simulink model "Demo_EP_IdleRandMerg"  (R2014a)
settings: Solver=FixedStepDiscrete  SolverMode=SingleTasking  StartTime=0.0  StopTime=inf  FixedStep=0.01  RelTol=1e-3
PostLoadFcn:
  | h_RPStest = RPStest;
model workspace (MAT data in the model file):
  gtest = 0
undefined symbols (not defined in the file or in its folder): avert, avert_freq_factor, avert_gaze_dirs_chance, avert_gaze_duration_factor, avert_head_frequency_factor, avert_head_speed, BML, BML1, BML2, bmlsL, bmlsM, bodyBusyFlag, clock, emotion_amount_factor, faceBusyFlag, fileID, GAZE_WIN, gazing, mut_freq_factor, mutual_gaze_duration_factor, P, pose_cat_chance, pose_chanc_factor, pose_chance_factor, pose_change_flag, pose_frequency_factor, pose_lean, pose_lean_flag, pose_speed, pose_twitch, pr, serial, STATE_BEFORE, STATE_GO, STATE_OVER, STATE_READY, Stateflow
libraries: simulink x24, instrumentlib x6, lib_affectiveChar_behavior x3, realtime_pacer_lib x2, lib_affectiveChar_input x1
(part 4 of 7)

== system Demo_EP_IdleRandMerg/GazeFollowSubsystem/resetGazeTarget/createGazePawn/sendSBM ==
  In2 : Inport  OutDataTypeStr=double  PortDimensions=[1000 1]
  f : TriggerPort  TriggerType=function-call
      settings: CopyFcn=Stateflow.SLINSF.SimulinkMan.removeBlockPreDeleteFcn  PreDeleteFcn=Stateflow.SLINSF.SimulinkMan.unsafePredeleteFcn
  C++ S-Function2 : S-Function  FunctionName=yarpSendText_sfun  Parameters='/sim/out/smb8', '/SB/in/sbm'  EnableBusSupport=off
  wires:
  In2/1 -> C++ S-Function2/1

== system Demo_EP_IdleRandMerg/facialExpr/facialExprGen/emotionBMLsLoop ==
  Amounts : Inport
  AUs : Inport  Port=2
  i : Inport  Port=3  OutMin=1  OutDataTypeStr=double
  e : Inport  Port=4
  Delay : Delay  DelayLength=10  InitialCondition=10
  For Iterator : ForIterator  IterationSource=external
  bml1 : M-S-Function  FunctionName=yarpSendText2_sfun  Parameters='/sim/out/bml9', '/SB/in/bml'
  displayBMLs : MATLAB Function  TreatAsAtomicUnit=on
  loopInBmls : MATLAB Function  TreatAsAtomicUnit=on
  wires:
  AUs/1 -> loopInBmls/2(arrAU)
  Amounts/1 -> loopInBmls/3(eAmount)
  loopInBmls/1(arrBML) -> Delay/1, displayBMLs/3(bml)
  e/1 -> displayBMLs/1(e)
  Delay/1 -> bml1/1
  i/1 -> loopInBmls/1(i), displayBMLs/2(i)

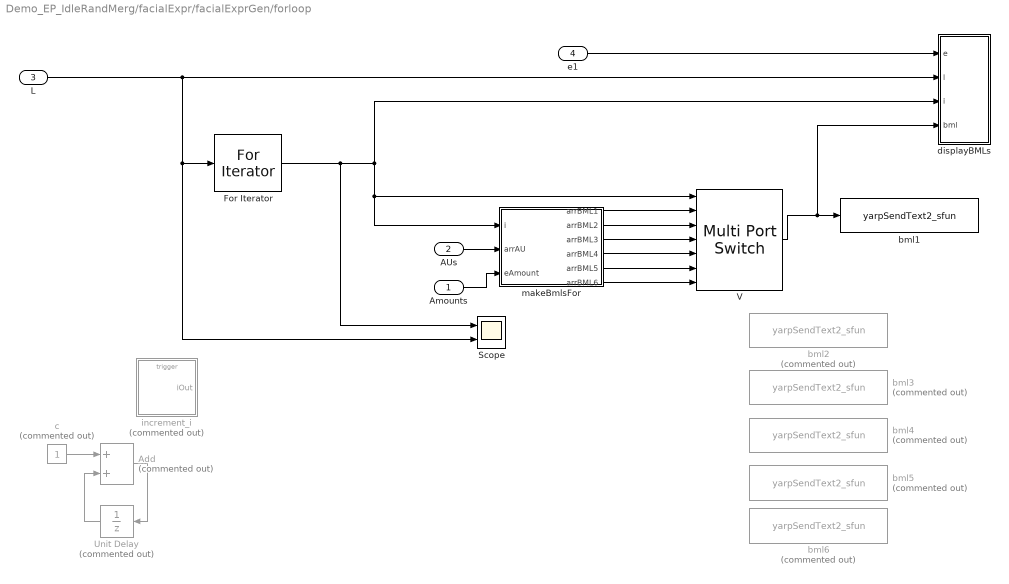
== system Demo_EP_IdleRandMerg/facialExpr/facialExprGen/forloop ==
  Amounts : Inport
  AUs : Inport  Port=2
  L : Inport  Port=3
  e1 : Inport  Port=4
  Add : Sum  Commented=on
  For Iterator : ForIterator  IterationSource=external  IterationVariableDataType=double
  Scope : Scope  NumInputPorts=2
      settings: YMin=3~3  YMax=3~3  SaveName=ScopeData7
  Unit Delay : UnitDelay  Commented=on  SampleTime=0.01
  V : MultiPortSwitch  Inputs=6
  bml1 : M-S-Function  FunctionName=yarpSendText2_sfun  Parameters='/sim/out/bml9', '/SB/in/bml'
  bml2 : M-S-Function  Commented=on  FunctionName=yarpSendText2_sfun  Parameters='/sim/out/bml10', '/SB/in/bml'
  bml3 : M-S-Function  Commented=on  FunctionName=yarpSendText2_sfun  Parameters='/sim/out/bml11', '/SB/in/bml'
  bml4 : M-S-Function  Commented=on  FunctionName=yarpSendText2_sfun  Parameters='/sim/out/bml12', '/SB/in/bml'
  bml5 : M-S-Function  Commented=on  FunctionName=yarpSendText2_sfun  Parameters='/sim/out/bml13', '/SB/in/bml'
  bml6 : M-S-Function  Commented=on  FunctionName=yarpSendText2_sfun  Parameters='/sim/out/bml14', '/SB/in/bml'
  c : Constant  Commented=on
  displayBMLs : MATLAB Function  TreatAsAtomicUnit=on
  increment_i : Subsystem  Commented=on
  makeBmlsFor : MATLAB Function  TreatAsAtomicUnit=on
  wires:
  L/1 -> Scope/2, For Iterator/1, displayBMLs/2(l)
  AUs/1 -> makeBmlsFor/2(arrAU)
  Amounts/1 -> makeBmlsFor/3(eAmount)
  e1/1 -> displayBMLs/1(e)
  Unit Delay/1 -> Add/2
  c/1 -> Add/1
  Add/1 -> Unit Delay/1
  For Iterator/1 -> Scope/1, V/1, makeBmlsFor/1(i), displayBMLs/3(i)
  V/1 -> displayBMLs/4(bml), bml1/1
  makeBmlsFor/1(arrBML1) -> V/2
  makeBmlsFor/2(arrBML2) -> V/3
  makeBmlsFor/3(arrBML3) -> V/4
  makeBmlsFor/4(arrBML4) -> V/5
  makeBmlsFor/5(arrBML5) -> V/6
  makeBmlsFor/6(arrBML6) -> V/7

== system Demo_EP_IdleRandMerg/facialExpr/facialExprGen/forloop1 ==
  Amounts : Inport
  AUs : Inport  Port=2
  L : Inport  Port=3
  e1 : Inport  Port=4
  Add : Sum  Commented=on
  Delay : Delay  DelayLength=50  InitialCondition=0
  For Iterator : ForIterator  IterationSource=external  IterationVariableDataType=double
  Scope : Scope  NumInputPorts=2
      settings: YMin=3~3  YMax=3~3  SaveName=ScopeData7
  Unit Delay : UnitDelay  Commented=on  SampleTime=0.01
  bml1 : M-S-Function  FunctionName=yarpSendText2_sfun  Parameters='/sim/out/bml9', '/SB/in/bml'
  c : Constant  Commented=on
  displayBMLs : MATLAB Function  TreatAsAtomicUnit=on
  increment_i : Subsystem  Commented=on
  makeBmls : MATLAB Function  TreatAsAtomicUnit=on
  wires:
  L/1 -> Scope/2, For Iterator/1, displayBMLs/2(l)
  AUs/1 -> makeBmls/2(arrAU)
  Amounts/1 -> makeBmls/3(eAmount)
  e1/1 -> displayBMLs/1(e)
  makeBmls/1(arrBML) -> Delay/1
  Unit Delay/1 -> Add/2
  c/1 -> Add/1
  Add/1 -> Unit Delay/1
  For Iterator/1 -> Scope/1, makeBmls/1(i), displayBMLs/3(i)
  Delay/1 -> displayBMLs/4(bml), bml1/1

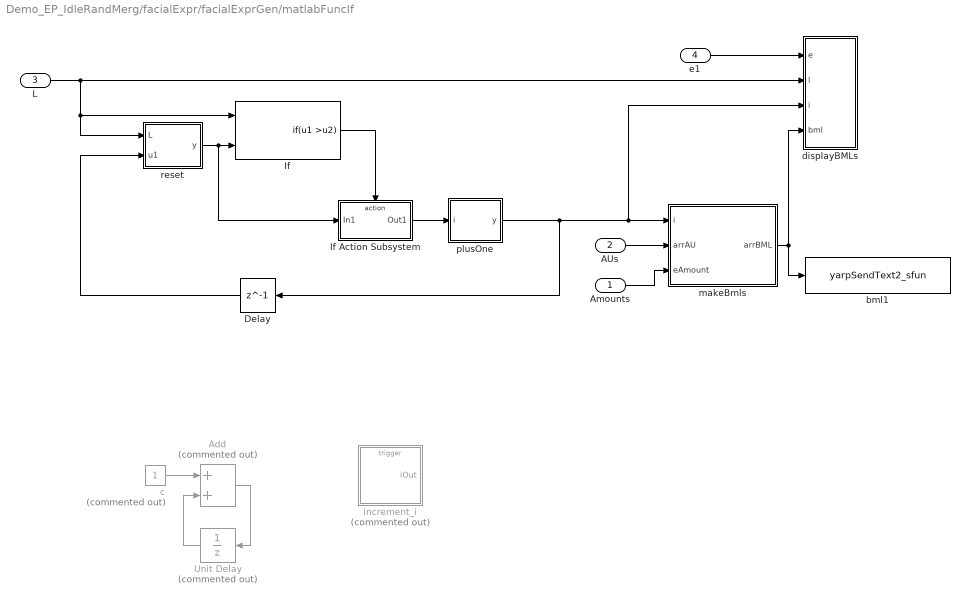
== system Demo_EP_IdleRandMerg/facialExpr/facialExprGen/matlabFuncIf ==
  Amounts : Inport
  AUs : Inport  Port=2
  L : Inport  Port=3
  e1 : Inport  Port=4
  Add : Sum  Commented=on
  Delay : Delay  DelayLength=1  InitialCondition=0
  If : If  NumInputs=2  IfExpression=u1 >u2  ShowElse=off
  If Action Subsystem : Subsystem  TreatAsAtomicUnit=on
  Unit Delay : UnitDelay  Commented=on  SampleTime=0.01
  bml1 : M-S-Function  FunctionName=yarpSendText2_sfun  Parameters='/sim/out/bml9', '/SB/in/bml'
  c : Constant  Commented=on
  displayBMLs : MATLAB Function  TreatAsAtomicUnit=on
  increment_i : Subsystem  Commented=on
  makeBmls : MATLAB Function  TreatAsAtomicUnit=on
  plusOne : MATLAB Function  TreatAsAtomicUnit=on
  reset : MATLAB Function  TreatAsAtomicUnit=on
  wires:
  L/1 -> reset/1(L), If/1, displayBMLs/2(l)
  AUs/1 -> makeBmls/2(arrAU)
  Amounts/1 -> makeBmls/3(eAmount)
  e1/1 -> displayBMLs/1(e)
  makeBmls/1(arrBML) -> displayBMLs/4(bml), bml1/1
  plusOne/1(y) -> Delay/1, displayBMLs/3(i), makeBmls/1(i)
  If/1 -> If Action Subsystem/Action
  Unit Delay/1 -> Add/2
  c/1 -> Add/1
  Add/1 -> Unit Delay/1
  If Action Subsystem/1(Out1) -> plusOne/1(i)
  Delay/1 -> reset/2(u1)
  reset/1(y) -> If Action Subsystem/1(In1), If/2

== system Demo_EP_IdleRandMerg/readGlove/normal glove/Normalize Index ==
  RawGlove : Inport
  Divide : Product  Inputs=*/  OutDataTypeStr=double  RndMeth=Nearest  InputSameDT=on
  Divide1 : Product  Inputs=**
  MinMax : Subsystem
  Range : Sum  Inputs=+-  OutDataTypeStr=double
  Ring1 : Constant  Value=100
  Subtract5 : Sum  Inputs=+-  OutDataTypeStr=double
  Norm100Out : Outport
  wires:
  MinMax/2(Max) -> Range/1
  Ring1/1 -> Divide1/2
  Subtract5/1 -> Divide/1
  MinMax/1(Min) -> Subtract5/2, Range/2
  RawGlove/1 -> Subtract5/1, MinMax/1(In1)
  Divide1/1 -> Norm100Out/1
  Divide/1 -> Divide1/1
  Range/1 -> Divide/2

== system Demo_EP_IdleRandMerg/readGlove/normal glove/Normalize Middle ==
  RawGlove : Inport
  Divide : Product  Inputs=*/  OutDataTypeStr=double  RndMeth=Nearest  InputSameDT=on
  Divide1 : Product  Inputs=**
  MinMax : Subsystem
  Range : Sum  Inputs=+-  OutDataTypeStr=double
  Ring1 : Constant  Value=100
  Subtract5 : Sum  Inputs=+-  OutDataTypeStr=double
  Norm100Out : Outport
  wires:
  MinMax/2(Max) -> Range/1
  Ring1/1 -> Divide1/2
  Subtract5/1 -> Divide/1
  MinMax/1(Min) -> Subtract5/2, Range/2
  RawGlove/1 -> Subtract5/1, MinMax/1(In1)
  Divide1/1 -> Norm100Out/1
  Divide/1 -> Divide1/1
  Range/1 -> Divide/2

== system Demo_EP_IdleRandMerg/readGlove/normal glove/Normalize Ring ==
  RawGlove : Inport
  Divide : Product  Inputs=*/  OutDataTypeStr=double  RndMeth=Nearest  InputSameDT=on
  Divide1 : Product  Inputs=**
  MinMax : Subsystem
  Range : Sum  Inputs=+-  OutDataTypeStr=double
  Ring1 : Constant  Value=100
  Subtract5 : Sum  Inputs=+-  OutDataTypeStr=double
  Norm100Out : Outport
  wires:
  MinMax/2(Max) -> Range/1
  Ring1/1 -> Divide1/2
  Subtract5/1 -> Divide/1
  MinMax/1(Min) -> Subtract5/2, Range/2
  RawGlove/1 -> Subtract5/1, MinMax/1(In1)
  Divide1/1 -> Norm100Out/1
  Divide/1 -> Divide1/1
  Range/1 -> Divide/2

== system Demo_EP_IdleRandMerg/facialExpr/facialExprGen/forloop/increment_i ==
  Trigger : TriggerPort  PortDimensions=1
  Add : Sum
  Scope : Scope  NumInputPorts=2
      settings: TimeRange=10  YMin=-5~-5  YMax=5~5  SaveName=ScopeData3
  Unit Delay : UnitDelay  SampleTime=0.01
  c : Constant
  iOut : Outport  OutMin=1  OutDataTypeStr=double  InitialOutput=1
  wires:
  Add/1 -> Scope/1, iOut/1, Unit Delay/1
  Unit Delay/1 -> Scope/2, Add/2
  c/1 -> Add/1

== system Demo_EP_IdleRandMerg/facialExpr/facialExprGen/forloop1/increment_i ==
  Trigger : TriggerPort  PortDimensions=1
  Add : Sum
  Scope : Scope  NumInputPorts=2
      settings: TimeRange=10  YMin=-5~-5  YMax=5~5  SaveName=ScopeData3
  Unit Delay : UnitDelay  SampleTime=0.01
  c : Constant
  iOut : Outport  OutMin=1  OutDataTypeStr=double  InitialOutput=1
  wires:
  Add/1 -> Scope/1, iOut/1, Unit Delay/1
  Unit Delay/1 -> Scope/2, Add/2
  c/1 -> Add/1

== system Demo_EP_IdleRandMerg/facialExpr/facialExprGen/matlabFuncIf/If Action Subsystem ==
  In1 : Inport
  Action Port : ActionPort  ActionType=then
  Scope : Scope
      settings: SaveName=ScopeData8
  Out1 : Outport
  wires:
  In1/1 -> Scope/1, Out1/1

== system Demo_EP_IdleRandMerg/facialExpr/facialExprGen/matlabFuncIf/increment_i ==
  Trigger : TriggerPort  PortDimensions=1
  Add : Sum
  Scope : Scope  NumInputPorts=2
      settings: TimeRange=10  YMin=-5~-5  YMax=5~5  SaveName=ScopeData3
  Unit Delay : UnitDelay  SampleTime=0.01
  c : Constant
  iOut : Outport  OutMin=1  OutDataTypeStr=double  InitialOutput=1
  wires:
  Add/1 -> Scope/1, iOut/1, Unit Delay/1
  Unit Delay/1 -> Scope/2, Add/2
  c/1 -> Add/1

== system Demo_EP_IdleRandMerg/readGlove/normal glove/Normalize Index/MinMax ==
  In1 : Inport
  Index1 : Constant  Value=0
  MinMax Running Resettable : simulink/Math Operations/MinMax Running Resettable  Function=min  vinit=100
  MinMax Running Resettable1 : simulink/Math Operations/MinMax Running Resettable  Function=max  vinit=0.0
  Min : Outport
  Max : Outport  Port=2
  wires:
  Index1/1 -> MinMax Running Resettable/2, MinMax Running Resettable1/2
  MinMax Running Resettable/1 -> Min/1
  In1/1 -> MinMax Running Resettable/1, MinMax Running Resettable1/1
  MinMax Running Resettable1/1 -> Max/1

== system Demo_EP_IdleRandMerg/readGlove/normal glove/Normalize Middle/MinMax ==
  In1 : Inport
  Index1 : Constant  Value=0
  MinMax Running Resettable : simulink/Math Operations/MinMax Running Resettable  Function=min  vinit=100
  MinMax Running Resettable1 : simulink/Math Operations/MinMax Running Resettable  Function=max  vinit=0.0
  Min : Outport
  Max : Outport  Port=2
  wires:
  Index1/1 -> MinMax Running Resettable/2, MinMax Running Resettable1/2
  MinMax Running Resettable/1 -> Min/1
  In1/1 -> MinMax Running Resettable/1, MinMax Running Resettable1/1
  MinMax Running Resettable1/1 -> Max/1

== system Demo_EP_IdleRandMerg/readGlove/normal glove/Normalize Ring/MinMax ==
  In1 : Inport
  Index1 : Constant  Value=0
  MinMax Running Resettable : simulink/Math Operations/MinMax Running Resettable  Function=min  vinit=100
  MinMax Running Resettable1 : simulink/Math Operations/MinMax Running Resettable  Function=max  vinit=0.0
  Min : Outport
  Max : Outport  Port=2
  wires:
  Index1/1 -> MinMax Running Resettable/2, MinMax Running Resettable1/2
  MinMax Running Resettable/1 -> Min/1
  In1/1 -> MinMax Running Resettable/1, MinMax Running Resettable1/1
  MinMax Running Resettable1/1 -> Max/1

== stateflow chart Demo_EP_IdleRandMerg/CharacterControl ==
  note: High Priority Tasks: Hand gesture for game
  state RPS_Scenario [parallel]
    settings: executionOrder=1
  note: Middle Priority Tasks: wave back at user and distance regulation
  state personalSpace_Controller [parallel]
    settings: executionOrder=5
  state wave_Controller [parallel]
    settings: executionOrder=7
  note: Low Priority Tasks: Idle gaze, pose and facial Expressions:
  state idlePose_Controller [parallel]
    settings: executionOrder=3
  state Gaze_Controller [parallel]
    settings: executionOrder=2
  state facialExpression_Controller [parallel]
    settings: executionOrder=4
  note: Parameters (can change
      | to seethe rangeof results)
      | -mutual_gaze_duration_factor
      | -avert_gaze_duration_factor
      | -avert_head_frequency_factor
      | -avert_head_speed(fast/slow/normal)
      | -avert_gaze_dirs_chance (down/up/normal)
      |
      | Inputs:(needed)
      | -faceAttendingFlag
      | -bodyAttendingFlag
  note: Parameters:
      | pose_selfAdaptor_chance_factor
      | pose_chance_factor
      | pose_frequency_factor
      | pose_speed(fast,slow,normal)
      | pose_lean(forward,backward,normal)
      |
      | Inputs:
      | -bodyAttendingFlag
  note: Parameters:
      |
      | Inputs:
      | -faceAttendingFlag
  note: Internal emotion/personality affects behavior modules (smile, gaze, pose)
  note: Instead of setting the factors directly in behavior or personality-emotion, added a module to centerlized and encapsulate all factors affecting behavior and their weights.
  state personality_Behavior_Factors [parallel]
    settings: executionOrder=9
  state emotion_Behavior_Factors [parallel]
    settings: executionOrder=10
  state custom_Behavior_Factors [parallel]
    settings: executionOrder=11
  note: Attention: if body or face is attending, no idle behavior are generated.
      | A queue is defined to priortize behaviors based on their importance.
  state attention_Controller [parallel]
    settings: executionOrder=8
  state sendBMLbyPriority [parallel]
    settings: executionOrder=6
    state sendH
      entry: BML=bmlsH(:,1);
      sendBML(BML);
      newBmlsH=removeQueue(bmlsH);
      bmlsH=newBmlsH;
    state init
      entry: n=encStr2Arr(' ');
      bmlsH=[n n n n n];
      bmlsM=[n n n n n];
      bmlsL=[n n n n n];
    state checkHighPriority
      entry:
      hEmpty=isEmptyQueue(bmlsH);
    state sendM
      entry: BML=bmlsM(:,1);
      sendBML(BML);
      newBmlsM= removeQueue(bmlsM);
      bmlsM=newBmlsM;
    state Mid
      entry:mEmpty=isEmptyQueue(bmlsM);
    state sendL
      entry: BML=bmlsL(:,1);
      sendBML(BML);
      newBmlsL= removeQueue(bmlsL);
      bmlsL=newBmlsL;
    state low
      entry:
      lEmpty=isEmptyQueue(bmlsL);
    note: Arrows' execution order is very importan here!
    state sendBML(In1) [function]
    sendH -> checkHighPriority
    checkHighPriority -> sendH [order 2] : [hEmpty~=1]
    (default) -> init
    init -> checkHighPriority
    checkHighPriority -> Mid [order 1] : [hEmpty==1]
    Mid -> checkHighPriority [order 4] : [mEmpty==1]
    sendM -> checkHighPriority [order 2]
    sendL -> checkHighPriority [order 3]
    low -> sendH [order 1] : [isEmptyQueue(bmlsH)~=1]
    Mid -> sendH [order 1] : [isEmptyQueue(bmlsH)~=1]
    sendM -> sendH [order 1] : [isEmptyQueue(bmlsH)~=1]
    sendL -> sendH [order 2] : [isEmptyQueue(bmlsH)~=1]
    Mid -> sendM [order 2] : [mEmpty~=1]
    Mid -> low [order 3] : [mEmpty==1]
    low -> Mid [order 4] : [lEmpty==1]
    low -> sendM [order 2] : [isEmptyQueue(bmlsM)~=1]
    sendL -> sendM [order 1] : [isEmptyQueue(bmlsM)~=1]
    low -> sendL [order 3] : [lEmpty~=1]
  data: In1 function_input double size=[1000 1]; bmls function_input; newBmls function_output; bmls function_input; empty function_output; emotion_amount_custom input double size=1; randArray input double size=[1,25]; poseArray input double size=[1,6]; gazeArray input double size=[1,6]; gameState output double size=1; inputUser input double size=1; bradHand output double size=1; userHand output double size=1; win output double size=1; temp local double size=1; diff local double size=1; uHand local double size=1; bHand local double size=1; bWinT output double size=1; uWinT output double size=1; randSmile local double size=1; boredom local double size=1; BOREDOM_THRESHOLD local double size=1; randAvertGazeChance local double size=1; randPoseChance local double size=1; interest local double size=1; r local double size=1; pa local double size=1; s local double size=1; randGazeDur local double size=1; P local double size=1 =0; smileN local double size=1; isSmiling input double size=1; body_isAttending input boolean size=1; face_isAttending input boolean size=1; avert local double size=1; GAZE_GUI local double size=1; GAZE_SOFTEYE local double size=1; GAZE_USER_HAND local double size=1; STATE_READY local double size=1 =0; STATE_GO local double size=1 =1; STATE_HAND local double size=1 =2; STATE_OVER local double size=1 =3; gazing local double size=1; GAZE_WIN local double size=1; randSlowPose local double size=1; STATE_BEFORE local double size=1 =4; STATE_RESULT local double size=1 =5; STATE_WAIT local double size=1 =6; HAPPY local double size=1 =4; SAD local double size=1 =4; CONTEMPT local double size=1 =4; BORED local double size=1 =4; FRUST local double size=1 =4; FEAR local double size=1 =4; IDLE local double size=1 =4; EXCITE local double size=1 =4; BML local double size=[1000,1]; pr local double size=1; t1 local; t2 local; round output double size=1; newBmlA local; fileID local double; xChangeFlag input boolean size=1; zChangeFlag input boolean size=1; isInvading input double size=1; inA input double size=1; handUp input double size=1; inV input double size=1; internalE input double size=1; personality input double size=1; BML2 local double size=[1000,1]; BML1 local double size=[1000,1]; t local double size=1; bodyBusyFlag local double size=1; n local double size=[1000,1]; bmlsL local double size=[1000,5]; hEmpty local double size=1; bmlsH local double size=[1000,5]; newBmlsH local double size=[1000,5]; newBmlsL local double size=[1000,5]; lEmpty local; newBmlsM local double size=[1000,5]; bmlsM local double size=[1000,5]; mEmpty local; avertH local double size=1; aChange input boolean size=1; vChange input boolean size=1; personalityChange input boolean size=1; faceBusyFlag local double size=1; personalityFlag input boolean size=1; vaFlag input boolean size=1; mutual_gaze_duration_factor local double size=1; avert_gaze_duration_factor local double size=1; avert_head_frequency_factor local double size=1; avert_gaze_dirs_chance local double size=1; avert_head_speed local double size=1; pose_chance_factor local double size=1; pose_cat_chance local double size=1; pose_frequency_factor local double size=1; pose_speed local double size=1; pose_lean local double size=1; pose_lean_flag local double size=1; pose_change_flag local double size=1; emotion_amount_factor local double size=[1,6]; avert_freq_factor local double size=1; mut_freq_factor local double size=1; pose_twitch local double size=1
  events: secs input RISING_EDGE_EVENT
  function newBmls=removeQueue(bmls):
    | function newBmls=removeQueue(bmls) 
    |     n=encStr2Arr(' ');
    |     newBmls=[n n n n n];
    |     newBmls(:,1)= bmls(:,2);
    |     newBmls(:,2)= bmls(:,3);
    |     newBmls(:,3)= bmls(:,4);
    |     newBmls(:,4)= bmls(:,5);
    |     newBmls(:,5)=encStr2Arr(' ');
  function empty=isEmptyQueue(bmls):
    | function empty=isEmptyQueue(bmls)
    | empty=1;
    | tempp=encStr2Arr(' ');
    | for i = 1:5
    |     if (isequal(bmls(:,i),tempp)==0)%there is a cell which is not equal to null
    |         empty=0;
    |         break
    |     end
    | end

== matlab function Demo_EP_IdleRandMerg/sendtoGUIFunction ==
  data: gameStatus input; bradHand input; userHand input; win input; bTotal input; uTotal input; gameNum input
function fcn(gameStatus, bradHand,userHand,win,bTotal,uTotal,gameNum)
%#codegen
setappdata(0,'gameStatus',gameStatus) 
setappdata(0,'bradHand',bradHand) 
setappdata(0,'userHand',userHand) 
setappdata(0,'win',win) 
setappdata(0,'uTotal',uTotal) 
setappdata(0,'bTotal',bTotal) 
setappdata(0,'gameNum',gameNum)

== matlab function Demo_EP_IdleRandMerg/readGlove/convertFunction ==
  data: u input; y output
function y = fcn(u)
%#codegen
%    paper=0; 'rock'=3;'scissors'=1;
%to 'paper'=1;'rock'=2;'scissors'=0;

if(u==0)
    u=1;
elseif(u==1)
    u=0;
elseif(u==3)
    u=2;
else 
    u=3;
end
y = u;
